simulink model "TST_CnvSet_Trq2Q"  (R2016b)
settings: Solver=FixedStepDiscrete  StartTime=0.0  StopTime=0.02  FixedStep=sampleTime  RelTol=1e-3
values from neighbouring files (symbols this model uses):
  testCase = 1    [initTST_CnvSet_Trq2Q_001.m]    (also in initTST_CnvSet_Trq2Q_002.m = 2; initTST_CnvSet_Trq2Q_003.m = 3)
libraries: simulink x31, UnitTest_Lib x27
settings Model: Creator=zhengjinyan  LastModifiedBy=zhengjinyan
settings DebuggingCC: SignalRangeChecking=error

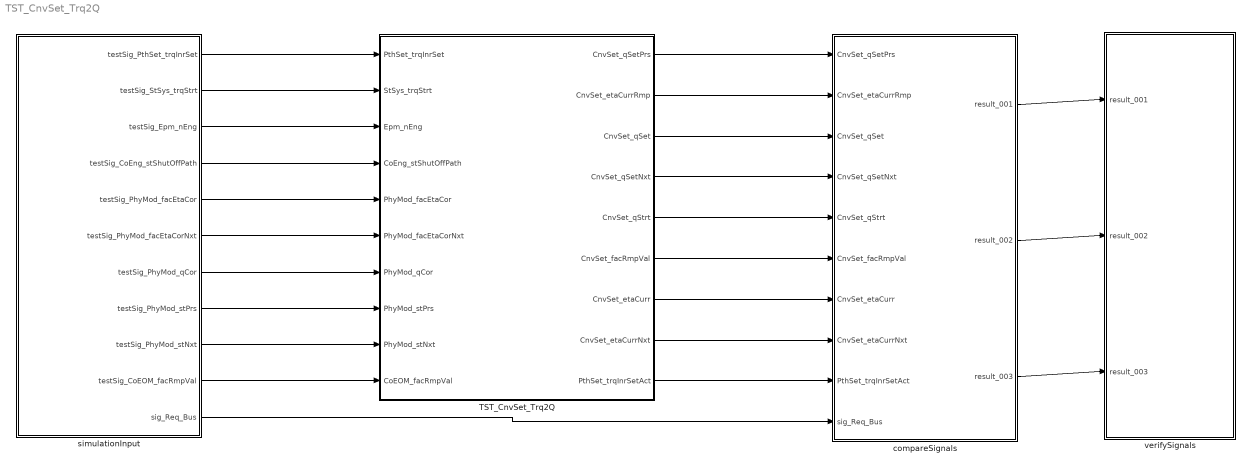
== system TST_CnvSet_Trq2Q ==
  TST_CnvSet_Trq2Q : Subsystem
  compareSignals : Subsystem
  simulationInput : Subsystem
  verifySignals : Subsystem
  wires:
  simulationInput/1(testSig_PthSet_trqInrSet) -> TST_CnvSet_Trq2Q/1(PthSet_trqInrSet)
  simulationInput/2(testSig_StSys_trqStrt) -> TST_CnvSet_Trq2Q/2(StSys_trqStrt)
  simulationInput/3(testSig_Epm_nEng) -> TST_CnvSet_Trq2Q/3(Epm_nEng)
  simulationInput/4(testSig_CoEng_stShutOffPath) -> TST_CnvSet_Trq2Q/4(CoEng_stShutOffPath)
  simulationInput/5(testSig_PhyMod_facEtaCor) -> TST_CnvSet_Trq2Q/5(PhyMod_facEtaCor)
  simulationInput/6(testSig_PhyMod_facEtaCorNxt) -> TST_CnvSet_Trq2Q/6(PhyMod_facEtaCorNxt)
  simulationInput/7(testSig_PhyMod_qCor) -> TST_CnvSet_Trq2Q/7(PhyMod_qCor)
  simulationInput/8(testSig_PhyMod_stPrs) -> TST_CnvSet_Trq2Q/8(PhyMod_stPrs)
  simulationInput/9(testSig_PhyMod_stNxt) -> TST_CnvSet_Trq2Q/9(PhyMod_stNxt)
  simulationInput/10(testSig_CoEOM_facRmpVal) -> TST_CnvSet_Trq2Q/10(CoEOM_facRmpVal)
  TST_CnvSet_Trq2Q/1(CnvSet_qSetPrs) -> compareSignals/1(CnvSet_qSetPrs)
  TST_CnvSet_Trq2Q/2(CnvSet_etaCurrRmp) -> compareSignals/2(CnvSet_etaCurrRmp)
  TST_CnvSet_Trq2Q/3(CnvSet_qSet) -> compareSignals/3(CnvSet_qSet)
  TST_CnvSet_Trq2Q/4(CnvSet_qSetNxt) -> compareSignals/4(CnvSet_qSetNxt)
  TST_CnvSet_Trq2Q/5(CnvSet_qStrt) -> compareSignals/5(CnvSet_qStrt)
  TST_CnvSet_Trq2Q/6(CnvSet_facRmpVal) -> compareSignals/6(CnvSet_facRmpVal)
  TST_CnvSet_Trq2Q/7(CnvSet_etaCurr) -> compareSignals/7(CnvSet_etaCurr)
  TST_CnvSet_Trq2Q/8(CnvSet_etaCurrNxt) -> compareSignals/8(CnvSet_etaCurrNxt)
  TST_CnvSet_Trq2Q/9(PthSet_trqInrSetAct) -> compareSignals/9(PthSet_trqInrSetAct)
  simulationInput/11(sig_Req_Bus) -> compareSignals/10(sig_Req_Bus)
  compareSignals/1(result_001) -> verifySignals/1(result_001)
  compareSignals/2(result_002) -> verifySignals/2(result_002)
  compareSignals/3(result_003) -> verifySignals/3(result_003)

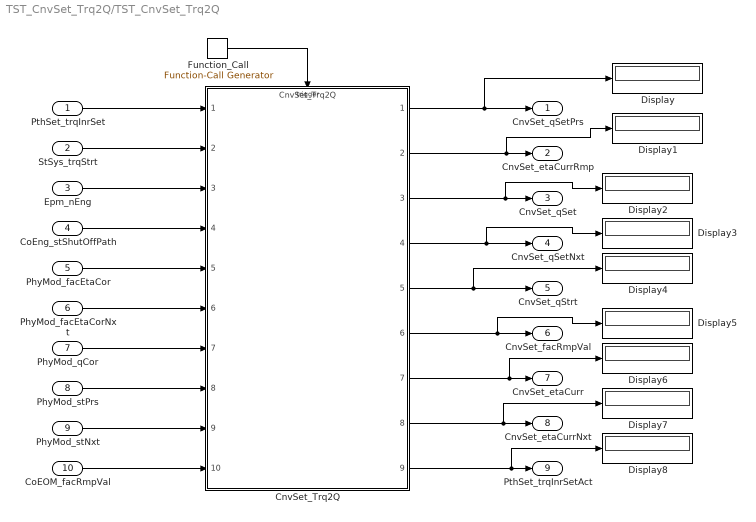
== system TST_CnvSet_Trq2Q/TST_CnvSet_Trq2Q ==
  PthSet_trqInrSet : Inport
  StSys_trqStrt : Inport  Port=2
  Epm_nEng : Inport  Port=3
  CoEng_stShutOffPath : Inport  Port=4
  PhyMod_facEtaCor : Inport  Port=5
  PhyMod_facEtaCorNxt : Inport  Port=6
  PhyMod_qCor : Inport  Port=7
  PhyMod_stPrs : Inport  Port=8
  PhyMod_stNxt : Inport  Port=9
  CoEOM_facRmpVal : Inport  Port=10
  CnvSet_Trq2Q : ModelReference  ModelNameDialog=CnvSet_Trq2Q  SimulationMode=Normal  ModelReferenceVersion=1.56  TriggerPortName=function  TriggerPortTriggerType=function-call  TriggerPortStatesWhenEnabling=held
  Display{,1..8} (9 alike) : Display
  Function_Call : simulink/Ports & Subsystems/Function-Call Generator  sample_time=sampleTime  numberOfIterations=1
  CnvSet_qSetPrs : Outport
  CnvSet_etaCurrRmp : Outport  Port=2
  CnvSet_qSet : Outport  Port=3
  CnvSet_qSetNxt : Outport  Port=4
  CnvSet_qStrt : Outport  Port=5
  CnvSet_facRmpVal : Outport  Port=6
  CnvSet_etaCurr : Outport  Port=7
  CnvSet_etaCurrNxt : Outport  Port=8
  PthSet_trqInrSetAct : Outport  Port=9
  wires:
  Function_Call/1 -> CnvSet_Trq2Q/Trigger
  PthSet_trqInrSet/1 -> CnvSet_Trq2Q/1
  StSys_trqStrt/1 -> CnvSet_Trq2Q/2
  Epm_nEng/1 -> CnvSet_Trq2Q/3
  CoEng_stShutOffPath/1 -> CnvSet_Trq2Q/4
  PhyMod_facEtaCor/1 -> CnvSet_Trq2Q/5
  PhyMod_facEtaCorNxt/1 -> CnvSet_Trq2Q/6
  PhyMod_qCor/1 -> CnvSet_Trq2Q/7
  PhyMod_stPrs/1 -> CnvSet_Trq2Q/8
  PhyMod_stNxt/1 -> CnvSet_Trq2Q/9
  CoEOM_facRmpVal/1 -> CnvSet_Trq2Q/10
  CnvSet_Trq2Q/1 -> Display/1, CnvSet_qSetPrs/1
  CnvSet_Trq2Q/2 -> Display1/1, CnvSet_etaCurrRmp/1
  CnvSet_Trq2Q/3 -> Display2/1, CnvSet_qSet/1
  CnvSet_Trq2Q/4 -> Display3/1, CnvSet_qSetNxt/1
  CnvSet_Trq2Q/5 -> Display4/1, CnvSet_qStrt/1
  CnvSet_Trq2Q/6 -> Display5/1, CnvSet_facRmpVal/1
  CnvSet_Trq2Q/7 -> Display6/1, CnvSet_etaCurr/1
  CnvSet_Trq2Q/9 -> Display8/1, PthSet_trqInrSetAct/1
  CnvSet_Trq2Q/8 -> Display7/1, CnvSet_etaCurrNxt/1

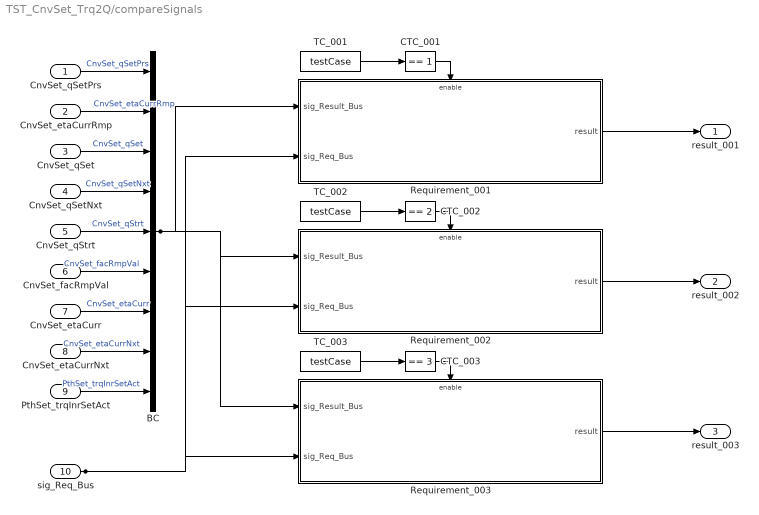
== system TST_CnvSet_Trq2Q/compareSignals ==
  CnvSet_qSetPrs : Inport
  CnvSet_etaCurrRmp : Inport  Port=2
  CnvSet_qSet : Inport  Port=3
  CnvSet_qSetNxt : Inport  Port=4
  CnvSet_qStrt : Inport  Port=5
  CnvSet_facRmpVal : Inport  Port=6
  CnvSet_etaCurr : Inport  Port=7
  CnvSet_etaCurrNxt : Inport  Port=8
  PthSet_trqInrSetAct : Inport  Port=9
  sig_Req_Bus : Inport  Port=10
  BC : BusCreator  Inputs=9
  CTC_001 : simulink/Logic and Bit Operations/Compare To Constant  relop===  const=1  OutDataTypeStr=boolean
  CTC_002 : simulink/Logic and Bit Operations/Compare To Constant  relop===  const=2  OutDataTypeStr=boolean
  CTC_003 : simulink/Logic and Bit Operations/Compare To Constant  relop===  const=3  OutDataTypeStr=boolean
  Requirement_001 : Subsystem
  Requirement_002 : Subsystem
  Requirement_003 : Subsystem
  TC_001 : Constant  Value=testCase
  TC_002 : Constant  Value=testCase
  TC_003 : Constant  Value=testCase
  result_001 : Outport
  result_002 : Outport  Port=2
  result_003 : Outport  Port=3
  wires:
  CnvSet_qSetPrs/1 -> BC/1  "CnvSet_qSetPrs"
  CnvSet_etaCurrRmp/1 -> BC/2  "CnvSet_etaCurrRmp"
  CnvSet_qSet/1 -> BC/3  "CnvSet_qSet"
  CnvSet_qSetNxt/1 -> BC/4  "CnvSet_qSetNxt"
  CnvSet_qStrt/1 -> BC/5  "CnvSet_qStrt"
  CnvSet_facRmpVal/1 -> BC/6  "CnvSet_facRmpVal"
  CnvSet_etaCurr/1 -> BC/7  "CnvSet_etaCurr"
  CnvSet_etaCurrNxt/1 -> BC/8  "CnvSet_etaCurrNxt"
  PthSet_trqInrSetAct/1 -> BC/9  "PthSet_trqInrSetAct"
  TC_001/1 -> CTC_001/1
  CTC_001/1 -> Requirement_001/Enable
  sig_Req_Bus/1 -> Requirement_001/2(sig_Req_Bus), Requirement_002/2(sig_Req_Bus), Requirement_003/2(sig_Req_Bus)
  BC/1 -> Requirement_001/1(sig_Result_Bus), Requirement_002/1(sig_Result_Bus), Requirement_003/1(sig_Result_Bus)
  Requirement_001/1(result) -> result_001/1
  TC_002/1 -> CTC_002/1
  CTC_002/1 -> Requirement_002/Enable
  Requirement_002/1(result) -> result_002/1
  TC_003/1 -> CTC_003/1
  CTC_003/1 -> Requirement_003/Enable
  Requirement_003/1(result) -> result_003/1

== system TST_CnvSet_Trq2Q/simulationInput ==
  BS : BusSelector  OutputSignals=testSig_PthSet_trqInrSet,testSig_StSys_trqStrt,testSig_Epm_nEng,testSig_CoEng_stShutOffPath,testSig_PhyMod_facEtaCor,testSig_PhyMod_facEtaCorNxt,testSig_PhyMod_qCor,testSig_PhyMod_stPrs,testSig_PhyMod_stNxt,testSig_CoEOM_facRmpVal
  MPSw : MultiPortSwitch  SaturateOnIntegerOverflow=on  InputSameDT=on
  TestCase : Constant  Value=testCase
  testSignals_R001 : Subsystem
  testSignals_R002 : Subsystem
  testSignals_R003 : Subsystem
  testSig_PthSet_trqInrSet : Outport
  testSig_StSys_trqStrt : Outport  Port=2
  testSig_Epm_nEng : Outport  Port=3
  testSig_CoEng_stShutOffPath : Outport  Port=4
  testSig_PhyMod_facEtaCor : Outport  Port=5
  testSig_PhyMod_facEtaCorNxt : Outport  Port=6
  testSig_PhyMod_qCor : Outport  Port=7
  testSig_PhyMod_stPrs : Outport  Port=8
  testSig_PhyMod_stNxt : Outport  Port=9
  testSig_CoEOM_facRmpVal : Outport  Port=10
  sig_Req_Bus : Outport  Port=11
  wires:
  BS/1 -> testSig_PthSet_trqInrSet/1  "<testSig_PthSet_trqInrSet>"
  BS/2 -> testSig_StSys_trqStrt/1  "<testSig_StSys_trqStrt>"
  BS/3 -> testSig_Epm_nEng/1  "<testSig_Epm_nEng>"
  BS/4 -> testSig_CoEng_stShutOffPath/1  "<testSig_CoEng_stShutOffPath>"
  BS/5 -> testSig_PhyMod_facEtaCor/1  "<testSig_PhyMod_facEtaCor>"
  BS/6 -> testSig_PhyMod_facEtaCorNxt/1  "<testSig_PhyMod_facEtaCorNxt>"
  BS/7 -> testSig_PhyMod_qCor/1  "<testSig_PhyMod_qCor>"
  BS/8 -> testSig_PhyMod_stPrs/1  "<testSig_PhyMod_stPrs>"
  BS/9 -> testSig_PhyMod_stNxt/1  "<testSig_PhyMod_stNxt>"
  BS/10 -> testSig_CoEOM_facRmpVal/1  "<testSig_CoEOM_facRmpVal>"
  MPSw/1 -> BS/1, sig_Req_Bus/1
  TestCase/1 -> MPSw/1
  testSignals_R001/1(testSignals) -> MPSw/2
  testSignals_R002/1(testSignals) -> MPSw/3
  testSignals_R003/1(testSignals) -> MPSw/4

== system TST_CnvSet_Trq2Q/verifySignals ==
  result_001 : Inport
  result_002 : Inport  Port=2
  result_003 : Inport  Port=3
  Assertion_001 : Assertion  Enabled=off
  Assertion_002 : Assertion  Enabled=off
  Assertion_003 : Assertion  Enabled=off
  wires:
  result_001/1 -> Assertion_001/1
  result_002/1 -> Assertion_002/1
  result_003/1 -> Assertion_003/1

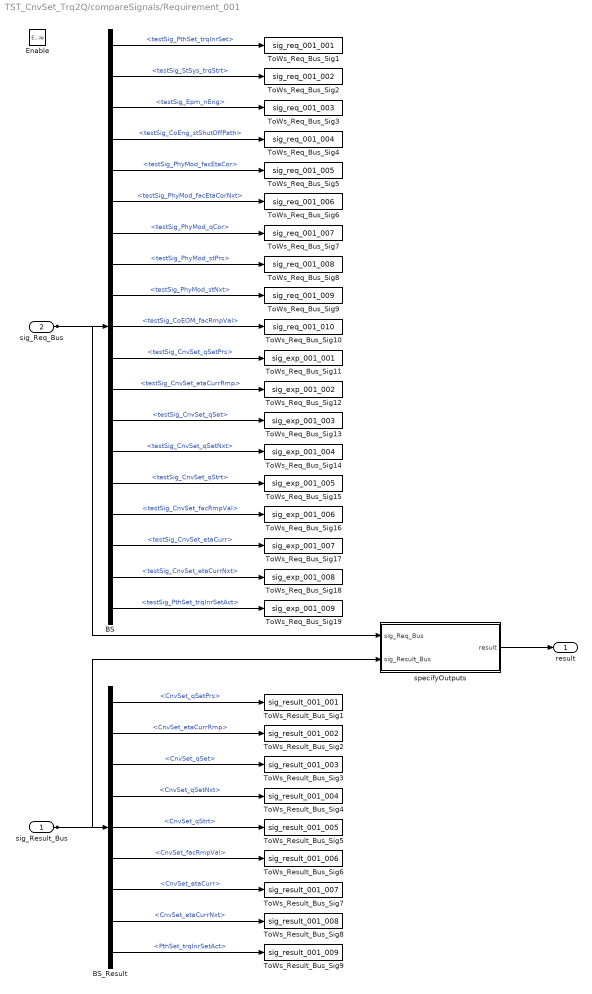
== system TST_CnvSet_Trq2Q/compareSignals/Requirement_001 ==
  sig_Result_Bus : Inport
  sig_Req_Bus : Inport  Port=2
  Enable : EnablePort
  BS : BusSelector  OutputSignals=testSig_PthSet_trqInrSet,testSig_StSys_trqStrt,testSig_Epm_nEng,testSig_CoEng_stShutOffPath,testSig_PhyMod_facEtaCor,testSig_PhyMod_facEtaCorNxt,testSig_PhyMod_qCor,testSig_PhyMod_stPrs,testSig_PhyMod_stNxt,testSig_CoEOM_facRmpVal,testSig_CnvSet_qSetPrs,testSig_CnvSet_etaCurrRmp,testSig_CnvSet_qSet,testSig_CnvSet_qSetNxt,testSig_CnvSet_qStrt,testSig_CnvSet_facRmpVal,testSig_CnvSet_etaCurr,testSig_CnvSet_etaCurrNxt,testSig_PthSet_trqInrSetAct
  BS_Result : BusSelector  OutputSignals=CnvSet_qSetPrs,CnvSet_etaCurrRmp,CnvSet_qSet,CnvSet_qSetNxt,CnvSet_qStrt,CnvSet_facRmpVal,CnvSet_etaCurr,CnvSet_etaCurrNxt,PthSet_trqInrSetAct
  ToWs_Req_Bus_Sig1 : ToWorkspace  VariableName=sig_req_001_001  SaveFormat=Structure With Time
  ToWs_Req_Bus_Sig10 : ToWorkspace  VariableName=sig_req_001_010  SaveFormat=Structure With Time
  ToWs_Req_Bus_Sig11 : ToWorkspace  VariableName=sig_exp_001_001  SaveFormat=Structure With Time
  ToWs_Req_Bus_Sig12 : ToWorkspace  VariableName=sig_exp_001_002  SaveFormat=Structure With Time
  ToWs_Req_Bus_Sig13 : ToWorkspace  VariableName=sig_exp_001_003  SaveFormat=Structure With Time
  ToWs_Req_Bus_Sig14 : ToWorkspace  VariableName=sig_exp_001_004  SaveFormat=Structure With Time
  ToWs_Req_Bus_Sig15 : ToWorkspace  VariableName=sig_exp_001_005  SaveFormat=Structure With Time
  ToWs_Req_Bus_Sig16 : ToWorkspace  VariableName=sig_exp_001_006  SaveFormat=Structure With Time
  ToWs_Req_Bus_Sig17 : ToWorkspace  VariableName=sig_exp_001_007  SaveFormat=Structure With Time
  ToWs_Req_Bus_Sig18 : ToWorkspace  VariableName=sig_exp_001_008  SaveFormat=Structure With Time
  ToWs_Req_Bus_Sig19 : ToWorkspace  VariableName=sig_exp_001_009  SaveFormat=Structure With Time
  ToWs_Req_Bus_Sig2 : ToWorkspace  VariableName=sig_req_001_002  SaveFormat=Structure With Time
  ToWs_Req_Bus_Sig3 : ToWorkspace  VariableName=sig_req_001_003  SaveFormat=Structure With Time
  ToWs_Req_Bus_Sig4 : ToWorkspace  VariableName=sig_req_001_004  SaveFormat=Structure With Time
  ToWs_Req_Bus_Sig5 : ToWorkspace  VariableName=sig_req_001_005  SaveFormat=Structure With Time
  ToWs_Req_Bus_Sig6 : ToWorkspace  VariableName=sig_req_001_006  SaveFormat=Structure With Time
  ToWs_Req_Bus_Sig7 : ToWorkspace  VariableName=sig_req_001_007  SaveFormat=Structure With Time
  ToWs_Req_Bus_Sig8 : ToWorkspace  VariableName=sig_req_001_008  SaveFormat=Structure With Time
  ToWs_Req_Bus_Sig9 : ToWorkspace  VariableName=sig_req_001_009  SaveFormat=Structure With Time
  ToWs_Result_Bus_Sig1 : ToWorkspace  VariableName=sig_result_001_001  SaveFormat=Structure With Time
  ToWs_Result_Bus_Sig2 : ToWorkspace  VariableName=sig_result_001_002  SaveFormat=Structure With Time
  ToWs_Result_Bus_Sig3 : ToWorkspace  VariableName=sig_result_001_003  SaveFormat=Structure With Time
  ToWs_Result_Bus_Sig4 : ToWorkspace  VariableName=sig_result_001_004  SaveFormat=Structure With Time
  ToWs_Result_Bus_Sig5 : ToWorkspace  VariableName=sig_result_001_005  SaveFormat=Structure With Time
  ToWs_Result_Bus_Sig6 : ToWorkspace  VariableName=sig_result_001_006  SaveFormat=Structure With Time
  ToWs_Result_Bus_Sig7 : ToWorkspace  VariableName=sig_result_001_007  SaveFormat=Structure With Time
  ToWs_Result_Bus_Sig8 : ToWorkspace  VariableName=sig_result_001_008  SaveFormat=Structure With Time
  ToWs_Result_Bus_Sig9 : ToWorkspace  VariableName=sig_result_001_009  SaveFormat=Structure With Time
  specifyOutputs : Subsystem
  result : Outport
  wires:
  sig_Req_Bus/1 -> BS/1, specifyOutputs/1(sig_Req_Bus)
  BS/1 -> ToWs_Req_Bus_Sig1/1  "<testSig_PthSet_trqInrSet>"
  BS/2 -> ToWs_Req_Bus_Sig2/1  "<testSig_StSys_trqStrt>"
  BS/3 -> ToWs_Req_Bus_Sig3/1  "<testSig_Epm_nEng>"
  BS/4 -> ToWs_Req_Bus_Sig4/1  "<testSig_CoEng_stShutOffPath>"
  BS/5 -> ToWs_Req_Bus_Sig5/1  "<testSig_PhyMod_facEtaCor>"
  BS/6 -> ToWs_Req_Bus_Sig6/1  "<testSig_PhyMod_facEtaCorNxt>"
  BS/7 -> ToWs_Req_Bus_Sig7/1  "<testSig_PhyMod_qCor>"
  BS/8 -> ToWs_Req_Bus_Sig8/1  "<testSig_PhyMod_stPrs>"
  BS/9 -> ToWs_Req_Bus_Sig9/1  "<testSig_PhyMod_stNxt>"
  BS/10 -> ToWs_Req_Bus_Sig10/1  "<testSig_CoEOM_facRmpVal>"
  BS/11 -> ToWs_Req_Bus_Sig11/1  "<testSig_CnvSet_qSetPrs>"
  BS/12 -> ToWs_Req_Bus_Sig12/1  "<testSig_CnvSet_etaCurrRmp>"
  BS/13 -> ToWs_Req_Bus_Sig13/1  "<testSig_CnvSet_qSet>"
  BS/14 -> ToWs_Req_Bus_Sig14/1  "<testSig_CnvSet_qSetNxt>"
  BS/15 -> ToWs_Req_Bus_Sig15/1  "<testSig_CnvSet_qStrt>"
  BS/16 -> ToWs_Req_Bus_Sig16/1  "<testSig_CnvSet_facRmpVal>"
  BS/17 -> ToWs_Req_Bus_Sig17/1  "<testSig_CnvSet_etaCurr>"
  BS/18 -> ToWs_Req_Bus_Sig18/1  "<testSig_CnvSet_etaCurrNxt>"
  BS/19 -> ToWs_Req_Bus_Sig19/1  "<testSig_PthSet_trqInrSetAct>"
  sig_Result_Bus/1 -> BS_Result/1, specifyOutputs/2(sig_Result_Bus)
  BS_Result/1 -> ToWs_Result_Bus_Sig1/1  "<CnvSet_qSetPrs>"
  BS_Result/2 -> ToWs_Result_Bus_Sig2/1  "<CnvSet_etaCurrRmp>"
  BS_Result/3 -> ToWs_Result_Bus_Sig3/1  "<CnvSet_qSet>"
  BS_Result/4 -> ToWs_Result_Bus_Sig4/1  "<CnvSet_qSetNxt>"
  BS_Result/5 -> ToWs_Result_Bus_Sig5/1  "<CnvSet_qStrt>"
  BS_Result/6 -> ToWs_Result_Bus_Sig6/1  "<CnvSet_facRmpVal>"
  BS_Result/7 -> ToWs_Result_Bus_Sig7/1  "<CnvSet_etaCurr>"
  BS_Result/8 -> ToWs_Result_Bus_Sig8/1  "<CnvSet_etaCurrNxt>"
  BS_Result/9 -> ToWs_Result_Bus_Sig9/1  "<PthSet_trqInrSetAct>"
  specifyOutputs/1(result) -> result/1

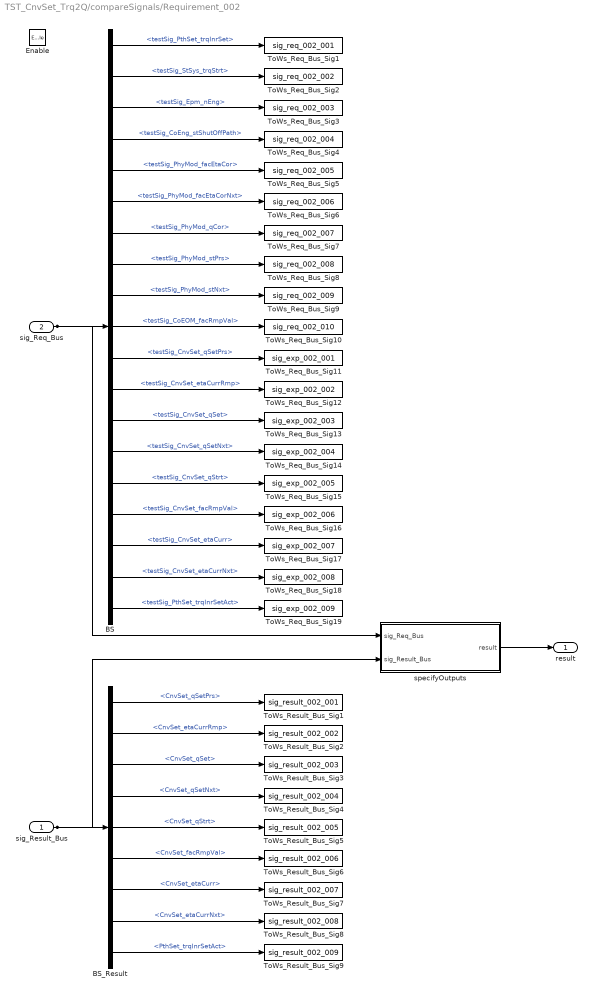
== system TST_CnvSet_Trq2Q/compareSignals/Requirement_002 ==
  sig_Result_Bus : Inport
  sig_Req_Bus : Inport  Port=2
  Enable : EnablePort
  BS : BusSelector  OutputSignals=testSig_PthSet_trqInrSet,testSig_StSys_trqStrt,testSig_Epm_nEng,testSig_CoEng_stShutOffPath,testSig_PhyMod_facEtaCor,testSig_PhyMod_facEtaCorNxt,testSig_PhyMod_qCor,testSig_PhyMod_stPrs,testSig_PhyMod_stNxt,testSig_CoEOM_facRmpVal,testSig_CnvSet_qSetPrs,testSig_CnvSet_etaCurrRmp,testSig_CnvSet_qSet,testSig_CnvSet_qSetNxt,testSig_CnvSet_qStrt,testSig_CnvSet_facRmpVal,testSig_CnvSet_etaCurr,testSig_CnvSet_etaCurrNxt,testSig_PthSet_trqInrSetAct
  BS_Result : BusSelector  OutputSignals=CnvSet_qSetPrs,CnvSet_etaCurrRmp,CnvSet_qSet,CnvSet_qSetNxt,CnvSet_qStrt,CnvSet_facRmpVal,CnvSet_etaCurr,CnvSet_etaCurrNxt,PthSet_trqInrSetAct
  ToWs_Req_Bus_Sig1 : ToWorkspace  VariableName=sig_req_002_001  SaveFormat=Structure With Time
  ToWs_Req_Bus_Sig10 : ToWorkspace  VariableName=sig_req_002_010  SaveFormat=Structure With Time
  ToWs_Req_Bus_Sig11 : ToWorkspace  VariableName=sig_exp_002_001  SaveFormat=Structure With Time
  ToWs_Req_Bus_Sig12 : ToWorkspace  VariableName=sig_exp_002_002  SaveFormat=Structure With Time
  ToWs_Req_Bus_Sig13 : ToWorkspace  VariableName=sig_exp_002_003  SaveFormat=Structure With Time
  ToWs_Req_Bus_Sig14 : ToWorkspace  VariableName=sig_exp_002_004  SaveFormat=Structure With Time
  ToWs_Req_Bus_Sig15 : ToWorkspace  VariableName=sig_exp_002_005  SaveFormat=Structure With Time
  ToWs_Req_Bus_Sig16 : ToWorkspace  VariableName=sig_exp_002_006  SaveFormat=Structure With Time
  ToWs_Req_Bus_Sig17 : ToWorkspace  VariableName=sig_exp_002_007  SaveFormat=Structure With Time
  ToWs_Req_Bus_Sig18 : ToWorkspace  VariableName=sig_exp_002_008  SaveFormat=Structure With Time
  ToWs_Req_Bus_Sig19 : ToWorkspace  VariableName=sig_exp_002_009  SaveFormat=Structure With Time
  ToWs_Req_Bus_Sig2 : ToWorkspace  VariableName=sig_req_002_002  SaveFormat=Structure With Time
  ToWs_Req_Bus_Sig3 : ToWorkspace  VariableName=sig_req_002_003  SaveFormat=Structure With Time
  ToWs_Req_Bus_Sig4 : ToWorkspace  VariableName=sig_req_002_004  SaveFormat=Structure With Time
  ToWs_Req_Bus_Sig5 : ToWorkspace  VariableName=sig_req_002_005  SaveFormat=Structure With Time
  ToWs_Req_Bus_Sig6 : ToWorkspace  VariableName=sig_req_002_006  SaveFormat=Structure With Time
  ToWs_Req_Bus_Sig7 : ToWorkspace  VariableName=sig_req_002_007  SaveFormat=Structure With Time
  ToWs_Req_Bus_Sig8 : ToWorkspace  VariableName=sig_req_002_008  SaveFormat=Structure With Time
  ToWs_Req_Bus_Sig9 : ToWorkspace  VariableName=sig_req_002_009  SaveFormat=Structure With Time
  ToWs_Result_Bus_Sig1 : ToWorkspace  VariableName=sig_result_002_001  SaveFormat=Structure With Time
  ToWs_Result_Bus_Sig2 : ToWorkspace  VariableName=sig_result_002_002  SaveFormat=Structure With Time
  ToWs_Result_Bus_Sig3 : ToWorkspace  VariableName=sig_result_002_003  SaveFormat=Structure With Time
  ToWs_Result_Bus_Sig4 : ToWorkspace  VariableName=sig_result_002_004  SaveFormat=Structure With Time
  ToWs_Result_Bus_Sig5 : ToWorkspace  VariableName=sig_result_002_005  SaveFormat=Structure With Time
  ToWs_Result_Bus_Sig6 : ToWorkspace  VariableName=sig_result_002_006  SaveFormat=Structure With Time
  ToWs_Result_Bus_Sig7 : ToWorkspace  VariableName=sig_result_002_007  SaveFormat=Structure With Time
  ToWs_Result_Bus_Sig8 : ToWorkspace  VariableName=sig_result_002_008  SaveFormat=Structure With Time
  ToWs_Result_Bus_Sig9 : ToWorkspace  VariableName=sig_result_002_009  SaveFormat=Structure With Time
  specifyOutputs : Subsystem
  result : Outport
  wires:
  sig_Req_Bus/1 -> BS/1, specifyOutputs/1(sig_Req_Bus)
  BS/1 -> ToWs_Req_Bus_Sig1/1  "<testSig_PthSet_trqInrSet>"
  BS/2 -> ToWs_Req_Bus_Sig2/1  "<testSig_StSys_trqStrt>"
  BS/3 -> ToWs_Req_Bus_Sig3/1  "<testSig_Epm_nEng>"
  BS/4 -> ToWs_Req_Bus_Sig4/1  "<testSig_CoEng_stShutOffPath>"
  BS/5 -> ToWs_Req_Bus_Sig5/1  "<testSig_PhyMod_facEtaCor>"
  BS/6 -> ToWs_Req_Bus_Sig6/1  "<testSig_PhyMod_facEtaCorNxt>"
  BS/7 -> ToWs_Req_Bus_Sig7/1  "<testSig_PhyMod_qCor>"
  BS/8 -> ToWs_Req_Bus_Sig8/1  "<testSig_PhyMod_stPrs>"
  BS/9 -> ToWs_Req_Bus_Sig9/1  "<testSig_PhyMod_stNxt>"
  BS/10 -> ToWs_Req_Bus_Sig10/1  "<testSig_CoEOM_facRmpVal>"
  BS/11 -> ToWs_Req_Bus_Sig11/1  "<testSig_CnvSet_qSetPrs>"
  BS/12 -> ToWs_Req_Bus_Sig12/1  "<testSig_CnvSet_etaCurrRmp>"
  BS/13 -> ToWs_Req_Bus_Sig13/1  "<testSig_CnvSet_qSet>"
  BS/14 -> ToWs_Req_Bus_Sig14/1  "<testSig_CnvSet_qSetNxt>"
  BS/15 -> ToWs_Req_Bus_Sig15/1  "<testSig_CnvSet_qStrt>"
  BS/16 -> ToWs_Req_Bus_Sig16/1  "<testSig_CnvSet_facRmpVal>"
  BS/17 -> ToWs_Req_Bus_Sig17/1  "<testSig_CnvSet_etaCurr>"
  BS/18 -> ToWs_Req_Bus_Sig18/1  "<testSig_CnvSet_etaCurrNxt>"
  BS/19 -> ToWs_Req_Bus_Sig19/1  "<testSig_PthSet_trqInrSetAct>"
  sig_Result_Bus/1 -> BS_Result/1, specifyOutputs/2(sig_Result_Bus)
  BS_Result/1 -> ToWs_Result_Bus_Sig1/1  "<CnvSet_qSetPrs>"
  BS_Result/2 -> ToWs_Result_Bus_Sig2/1  "<CnvSet_etaCurrRmp>"
  BS_Result/3 -> ToWs_Result_Bus_Sig3/1  "<CnvSet_qSet>"
  BS_Result/4 -> ToWs_Result_Bus_Sig4/1  "<CnvSet_qSetNxt>"
  BS_Result/5 -> ToWs_Result_Bus_Sig5/1  "<CnvSet_qStrt>"
  BS_Result/6 -> ToWs_Result_Bus_Sig6/1  "<CnvSet_facRmpVal>"
  BS_Result/7 -> ToWs_Result_Bus_Sig7/1  "<CnvSet_etaCurr>"
  BS_Result/8 -> ToWs_Result_Bus_Sig8/1  "<CnvSet_etaCurrNxt>"
  BS_Result/9 -> ToWs_Result_Bus_Sig9/1  "<PthSet_trqInrSetAct>"
  specifyOutputs/1(result) -> result/1

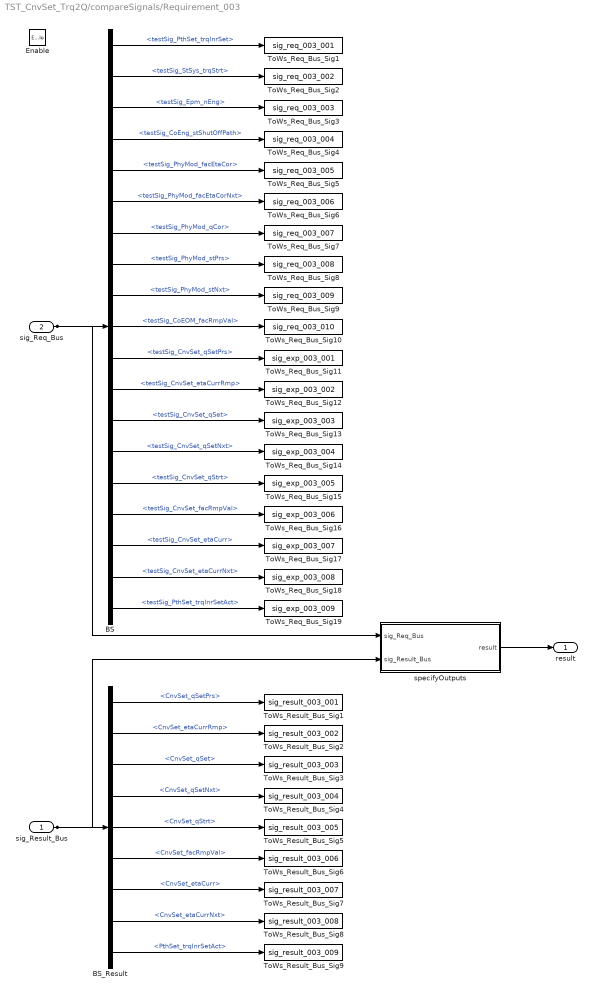
== system TST_CnvSet_Trq2Q/compareSignals/Requirement_003 ==
  sig_Result_Bus : Inport
  sig_Req_Bus : Inport  Port=2
  Enable : EnablePort
  BS : BusSelector  OutputSignals=testSig_PthSet_trqInrSet,testSig_StSys_trqStrt,testSig_Epm_nEng,testSig_CoEng_stShutOffPath,testSig_PhyMod_facEtaCor,testSig_PhyMod_facEtaCorNxt,testSig_PhyMod_qCor,testSig_PhyMod_stPrs,testSig_PhyMod_stNxt,testSig_CoEOM_facRmpVal,testSig_CnvSet_qSetPrs,testSig_CnvSet_etaCurrRmp,testSig_CnvSet_qSet,testSig_CnvSet_qSetNxt,testSig_CnvSet_qStrt,testSig_CnvSet_facRmpVal,testSig_CnvSet_etaCurr,testSig_CnvSet_etaCurrNxt,testSig_PthSet_trqInrSetAct
  BS_Result : BusSelector  OutputSignals=CnvSet_qSetPrs,CnvSet_etaCurrRmp,CnvSet_qSet,CnvSet_qSetNxt,CnvSet_qStrt,CnvSet_facRmpVal,CnvSet_etaCurr,CnvSet_etaCurrNxt,PthSet_trqInrSetAct
  ToWs_Req_Bus_Sig1 : ToWorkspace  VariableName=sig_req_003_001  SaveFormat=Structure With Time
  ToWs_Req_Bus_Sig10 : ToWorkspace  VariableName=sig_req_003_010  SaveFormat=Structure With Time
  ToWs_Req_Bus_Sig11 : ToWorkspace  VariableName=sig_exp_003_001  SaveFormat=Structure With Time
  ToWs_Req_Bus_Sig12 : ToWorkspace  VariableName=sig_exp_003_002  SaveFormat=Structure With Time
  ToWs_Req_Bus_Sig13 : ToWorkspace  VariableName=sig_exp_003_003  SaveFormat=Structure With Time
  ToWs_Req_Bus_Sig14 : ToWorkspace  VariableName=sig_exp_003_004  SaveFormat=Structure With Time
  ToWs_Req_Bus_Sig15 : ToWorkspace  VariableName=sig_exp_003_005  SaveFormat=Structure With Time
  ToWs_Req_Bus_Sig16 : ToWorkspace  VariableName=sig_exp_003_006  SaveFormat=Structure With Time
  ToWs_Req_Bus_Sig17 : ToWorkspace  VariableName=sig_exp_003_007  SaveFormat=Structure With Time
  ToWs_Req_Bus_Sig18 : ToWorkspace  VariableName=sig_exp_003_008  SaveFormat=Structure With Time
  ToWs_Req_Bus_Sig19 : ToWorkspace  VariableName=sig_exp_003_009  SaveFormat=Structure With Time
  ToWs_Req_Bus_Sig2 : ToWorkspace  VariableName=sig_req_003_002  SaveFormat=Structure With Time
  ToWs_Req_Bus_Sig3 : ToWorkspace  VariableName=sig_req_003_003  SaveFormat=Structure With Time
  ToWs_Req_Bus_Sig4 : ToWorkspace  VariableName=sig_req_003_004  SaveFormat=Structure With Time
  ToWs_Req_Bus_Sig5 : ToWorkspace  VariableName=sig_req_003_005  SaveFormat=Structure With Time
  ToWs_Req_Bus_Sig6 : ToWorkspace  VariableName=sig_req_003_006  SaveFormat=Structure With Time
  ToWs_Req_Bus_Sig7 : ToWorkspace  VariableName=sig_req_003_007  SaveFormat=Structure With Time
  ToWs_Req_Bus_Sig8 : ToWorkspace  VariableName=sig_req_003_008  SaveFormat=Structure With Time
  ToWs_Req_Bus_Sig9 : ToWorkspace  VariableName=sig_req_003_009  SaveFormat=Structure With Time
  ToWs_Result_Bus_Sig1 : ToWorkspace  VariableName=sig_result_003_001  SaveFormat=Structure With Time
  ToWs_Result_Bus_Sig2 : ToWorkspace  VariableName=sig_result_003_002  SaveFormat=Structure With Time
  ToWs_Result_Bus_Sig3 : ToWorkspace  VariableName=sig_result_003_003  SaveFormat=Structure With Time
  ToWs_Result_Bus_Sig4 : ToWorkspace  VariableName=sig_result_003_004  SaveFormat=Structure With Time
  ToWs_Result_Bus_Sig5 : ToWorkspace  VariableName=sig_result_003_005  SaveFormat=Structure With Time
  ToWs_Result_Bus_Sig6 : ToWorkspace  VariableName=sig_result_003_006  SaveFormat=Structure With Time
  ToWs_Result_Bus_Sig7 : ToWorkspace  VariableName=sig_result_003_007  SaveFormat=Structure With Time
  ToWs_Result_Bus_Sig8 : ToWorkspace  VariableName=sig_result_003_008  SaveFormat=Structure With Time
  ToWs_Result_Bus_Sig9 : ToWorkspace  VariableName=sig_result_003_009  SaveFormat=Structure With Time
  specifyOutputs : Subsystem
  result : Outport
  wires:
  sig_Req_Bus/1 -> BS/1, specifyOutputs/1(sig_Req_Bus)
  BS/1 -> ToWs_Req_Bus_Sig1/1  "<testSig_PthSet_trqInrSet>"
  BS/2 -> ToWs_Req_Bus_Sig2/1  "<testSig_StSys_trqStrt>"
  BS/3 -> ToWs_Req_Bus_Sig3/1  "<testSig_Epm_nEng>"
  BS/4 -> ToWs_Req_Bus_Sig4/1  "<testSig_CoEng_stShutOffPath>"
  BS/5 -> ToWs_Req_Bus_Sig5/1  "<testSig_PhyMod_facEtaCor>"
  BS/6 -> ToWs_Req_Bus_Sig6/1  "<testSig_PhyMod_facEtaCorNxt>"
  BS/7 -> ToWs_Req_Bus_Sig7/1  "<testSig_PhyMod_qCor>"
  BS/8 -> ToWs_Req_Bus_Sig8/1  "<testSig_PhyMod_stPrs>"
  BS/9 -> ToWs_Req_Bus_Sig9/1  "<testSig_PhyMod_stNxt>"
  BS/10 -> ToWs_Req_Bus_Sig10/1  "<testSig_CoEOM_facRmpVal>"
  BS/11 -> ToWs_Req_Bus_Sig11/1  "<testSig_CnvSet_qSetPrs>"
  BS/12 -> ToWs_Req_Bus_Sig12/1  "<testSig_CnvSet_etaCurrRmp>"
  BS/13 -> ToWs_Req_Bus_Sig13/1  "<testSig_CnvSet_qSet>"
  BS/14 -> ToWs_Req_Bus_Sig14/1  "<testSig_CnvSet_qSetNxt>"
  BS/15 -> ToWs_Req_Bus_Sig15/1  "<testSig_CnvSet_qStrt>"
  BS/16 -> ToWs_Req_Bus_Sig16/1  "<testSig_CnvSet_facRmpVal>"
  BS/17 -> ToWs_Req_Bus_Sig17/1  "<testSig_CnvSet_etaCurr>"
  BS/18 -> ToWs_Req_Bus_Sig18/1  "<testSig_CnvSet_etaCurrNxt>"
  BS/19 -> ToWs_Req_Bus_Sig19/1  "<testSig_PthSet_trqInrSetAct>"
  sig_Result_Bus/1 -> BS_Result/1, specifyOutputs/2(sig_Result_Bus)
  BS_Result/1 -> ToWs_Result_Bus_Sig1/1  "<CnvSet_qSetPrs>"
  BS_Result/2 -> ToWs_Result_Bus_Sig2/1  "<CnvSet_etaCurrRmp>"
  BS_Result/3 -> ToWs_Result_Bus_Sig3/1  "<CnvSet_qSet>"
  BS_Result/4 -> ToWs_Result_Bus_Sig4/1  "<CnvSet_qSetNxt>"
  BS_Result/5 -> ToWs_Result_Bus_Sig5/1  "<CnvSet_qStrt>"
  BS_Result/6 -> ToWs_Result_Bus_Sig6/1  "<CnvSet_facRmpVal>"
  BS_Result/7 -> ToWs_Result_Bus_Sig7/1  "<CnvSet_etaCurr>"
  BS_Result/8 -> ToWs_Result_Bus_Sig8/1  "<CnvSet_etaCurrNxt>"
  BS_Result/9 -> ToWs_Result_Bus_Sig9/1  "<PthSet_trqInrSetAct>"
  specifyOutputs/1(result) -> result/1

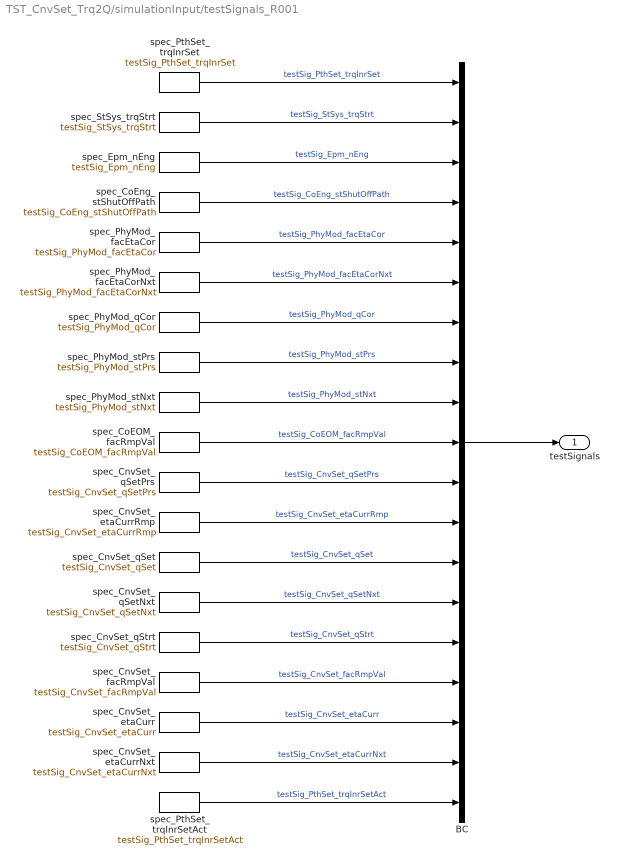
== system TST_CnvSet_Trq2Q/simulationInput/testSignals_R001 ==
  BC : BusCreator  Inputs=19
  spec_CnvSet_etaCurr : FromWorkspace  VariableName=testSig_CnvSet_etaCurr  Interpolate=off  OutputAfterFinalValue=Holding final value
  spec_CnvSet_etaCurrNxt : FromWorkspace  VariableName=testSig_CnvSet_etaCurrNxt  Interpolate=off  OutputAfterFinalValue=Holding final value
  spec_CnvSet_etaCurrRmp : FromWorkspace  VariableName=testSig_CnvSet_etaCurrRmp  Interpolate=off  OutputAfterFinalValue=Holding final value
  spec_CnvSet_facRmpVal : FromWorkspace  VariableName=testSig_CnvSet_facRmpVal  Interpolate=off  OutputAfterFinalValue=Holding final value
  spec_CnvSet_qSet : FromWorkspace  VariableName=testSig_CnvSet_qSet  Interpolate=off  OutputAfterFinalValue=Holding final value
  spec_CnvSet_qSetNxt : FromWorkspace  VariableName=testSig_CnvSet_qSetNxt  Interpolate=off  OutputAfterFinalValue=Holding final value
  spec_CnvSet_qSetPrs : FromWorkspace  VariableName=testSig_CnvSet_qSetPrs  Interpolate=off  OutputAfterFinalValue=Holding final value
  spec_CnvSet_qStrt : FromWorkspace  VariableName=testSig_CnvSet_qStrt  Interpolate=off  OutputAfterFinalValue=Holding final value
  spec_CoEOM_facRmpVal : FromWorkspace  VariableName=testSig_CoEOM_facRmpVal  Interpolate=off  OutputAfterFinalValue=Holding final value
  spec_CoEng_stShutOffPath : FromWorkspace  VariableName=testSig_CoEng_stShutOffPath  Interpolate=off  OutputAfterFinalValue=Holding final value
  spec_Epm_nEng : FromWorkspace  VariableName=testSig_Epm_nEng  Interpolate=off  OutputAfterFinalValue=Holding final value
  spec_PhyMod_facEtaCor : FromWorkspace  VariableName=testSig_PhyMod_facEtaCor  Interpolate=off  OutputAfterFinalValue=Holding final value
  spec_PhyMod_facEtaCorNxt : FromWorkspace  VariableName=testSig_PhyMod_facEtaCorNxt  Interpolate=off  OutputAfterFinalValue=Holding final value
  spec_PhyMod_qCor : FromWorkspace  VariableName=testSig_PhyMod_qCor  Interpolate=off  OutputAfterFinalValue=Holding final value
  spec_PhyMod_stNxt : FromWorkspace  VariableName=testSig_PhyMod_stNxt  Interpolate=off  OutputAfterFinalValue=Holding final value
  spec_PhyMod_stPrs : FromWorkspace  VariableName=testSig_PhyMod_stPrs  Interpolate=off  OutputAfterFinalValue=Holding final value
  spec_PthSet_trqInrSet : FromWorkspace  VariableName=testSig_PthSet_trqInrSet  Interpolate=off  OutputAfterFinalValue=Holding final value
  spec_PthSet_trqInrSetAct : FromWorkspace  VariableName=testSig_PthSet_trqInrSetAct  Interpolate=off  OutputAfterFinalValue=Holding final value
  spec_StSys_trqStrt : FromWorkspace  VariableName=testSig_StSys_trqStrt  Interpolate=off  OutputAfterFinalValue=Holding final value
  testSignals : Outport
  wires:
  BC/1 -> testSignals/1
  spec_PthSet_trqInrSet/1 -> BC/1  "testSig_PthSet_trqInrSet"
  spec_StSys_trqStrt/1 -> BC/2  "testSig_StSys_trqStrt"
  spec_Epm_nEng/1 -> BC/3  "testSig_Epm_nEng"
  spec_CoEng_stShutOffPath/1 -> BC/4  "testSig_CoEng_stShutOffPath"
  spec_PhyMod_facEtaCor/1 -> BC/5  "testSig_PhyMod_facEtaCor"
  spec_PhyMod_facEtaCorNxt/1 -> BC/6  "testSig_PhyMod_facEtaCorNxt"
  spec_PhyMod_qCor/1 -> BC/7  "testSig_PhyMod_qCor"
  spec_PhyMod_stPrs/1 -> BC/8  "testSig_PhyMod_stPrs"
  spec_PhyMod_stNxt/1 -> BC/9  "testSig_PhyMod_stNxt"
  spec_CoEOM_facRmpVal/1 -> BC/10  "testSig_CoEOM_facRmpVal"
  spec_CnvSet_qSetPrs/1 -> BC/11  "testSig_CnvSet_qSetPrs"
  spec_CnvSet_etaCurrRmp/1 -> BC/12  "testSig_CnvSet_etaCurrRmp"
  spec_CnvSet_qSet/1 -> BC/13  "testSig_CnvSet_qSet"
  spec_CnvSet_qSetNxt/1 -> BC/14  "testSig_CnvSet_qSetNxt"
  spec_CnvSet_qStrt/1 -> BC/15  "testSig_CnvSet_qStrt"
  spec_CnvSet_facRmpVal/1 -> BC/16  "testSig_CnvSet_facRmpVal"
  spec_CnvSet_etaCurr/1 -> BC/17  "testSig_CnvSet_etaCurr"
  spec_CnvSet_etaCurrNxt/1 -> BC/18  "testSig_CnvSet_etaCurrNxt"
  spec_PthSet_trqInrSetAct/1 -> BC/19  "testSig_PthSet_trqInrSetAct"

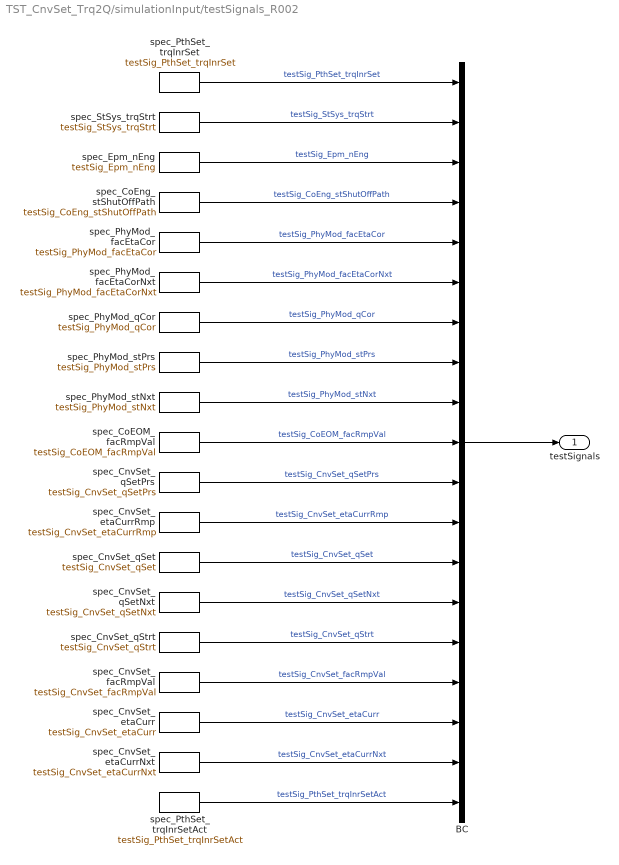
== system TST_CnvSet_Trq2Q/simulationInput/testSignals_R002 ==
  BC : BusCreator  Inputs=19
  spec_CnvSet_etaCurr : FromWorkspace  VariableName=testSig_CnvSet_etaCurr  Interpolate=off  OutputAfterFinalValue=Holding final value
  spec_CnvSet_etaCurrNxt : FromWorkspace  VariableName=testSig_CnvSet_etaCurrNxt  Interpolate=off  OutputAfterFinalValue=Holding final value
  spec_CnvSet_etaCurrRmp : FromWorkspace  VariableName=testSig_CnvSet_etaCurrRmp  Interpolate=off  OutputAfterFinalValue=Holding final value
  spec_CnvSet_facRmpVal : FromWorkspace  VariableName=testSig_CnvSet_facRmpVal  Interpolate=off  OutputAfterFinalValue=Holding final value
  spec_CnvSet_qSet : FromWorkspace  VariableName=testSig_CnvSet_qSet  Interpolate=off  OutputAfterFinalValue=Holding final value
  spec_CnvSet_qSetNxt : FromWorkspace  VariableName=testSig_CnvSet_qSetNxt  Interpolate=off  OutputAfterFinalValue=Holding final value
  spec_CnvSet_qSetPrs : FromWorkspace  VariableName=testSig_CnvSet_qSetPrs  Interpolate=off  OutputAfterFinalValue=Holding final value
  spec_CnvSet_qStrt : FromWorkspace  VariableName=testSig_CnvSet_qStrt  Interpolate=off  OutputAfterFinalValue=Holding final value
  spec_CoEOM_facRmpVal : FromWorkspace  VariableName=testSig_CoEOM_facRmpVal  Interpolate=off  OutputAfterFinalValue=Holding final value
  spec_CoEng_stShutOffPath : FromWorkspace  VariableName=testSig_CoEng_stShutOffPath  Interpolate=off  OutputAfterFinalValue=Holding final value
  spec_Epm_nEng : FromWorkspace  VariableName=testSig_Epm_nEng  Interpolate=off  OutputAfterFinalValue=Holding final value
  spec_PhyMod_facEtaCor : FromWorkspace  VariableName=testSig_PhyMod_facEtaCor  Interpolate=off  OutputAfterFinalValue=Holding final value
  spec_PhyMod_facEtaCorNxt : FromWorkspace  VariableName=testSig_PhyMod_facEtaCorNxt  Interpolate=off  OutputAfterFinalValue=Holding final value
  spec_PhyMod_qCor : FromWorkspace  VariableName=testSig_PhyMod_qCor  Interpolate=off  OutputAfterFinalValue=Holding final value
  spec_PhyMod_stNxt : FromWorkspace  VariableName=testSig_PhyMod_stNxt  Interpolate=off  OutputAfterFinalValue=Holding final value
  spec_PhyMod_stPrs : FromWorkspace  VariableName=testSig_PhyMod_stPrs  Interpolate=off  OutputAfterFinalValue=Holding final value
  spec_PthSet_trqInrSet : FromWorkspace  VariableName=testSig_PthSet_trqInrSet  Interpolate=off  OutputAfterFinalValue=Holding final value
  spec_PthSet_trqInrSetAct : FromWorkspace  VariableName=testSig_PthSet_trqInrSetAct  Interpolate=off  OutputAfterFinalValue=Holding final value
  spec_StSys_trqStrt : FromWorkspace  VariableName=testSig_StSys_trqStrt  Interpolate=off  OutputAfterFinalValue=Holding final value
  testSignals : Outport
  wires:
  BC/1 -> testSignals/1
  spec_PthSet_trqInrSet/1 -> BC/1  "testSig_PthSet_trqInrSet"
  spec_StSys_trqStrt/1 -> BC/2  "testSig_StSys_trqStrt"
  spec_Epm_nEng/1 -> BC/3  "testSig_Epm_nEng"
  spec_CoEng_stShutOffPath/1 -> BC/4  "testSig_CoEng_stShutOffPath"
  spec_PhyMod_facEtaCor/1 -> BC/5  "testSig_PhyMod_facEtaCor"
  spec_PhyMod_facEtaCorNxt/1 -> BC/6  "testSig_PhyMod_facEtaCorNxt"
  spec_PhyMod_qCor/1 -> BC/7  "testSig_PhyMod_qCor"
  spec_PhyMod_stPrs/1 -> BC/8  "testSig_PhyMod_stPrs"
  spec_PhyMod_stNxt/1 -> BC/9  "testSig_PhyMod_stNxt"
  spec_CoEOM_facRmpVal/1 -> BC/10  "testSig_CoEOM_facRmpVal"
  spec_CnvSet_qSetPrs/1 -> BC/11  "testSig_CnvSet_qSetPrs"
  spec_CnvSet_etaCurrRmp/1 -> BC/12  "testSig_CnvSet_etaCurrRmp"
  spec_CnvSet_qSet/1 -> BC/13  "testSig_CnvSet_qSet"
  spec_CnvSet_qSetNxt/1 -> BC/14  "testSig_CnvSet_qSetNxt"
  spec_CnvSet_qStrt/1 -> BC/15  "testSig_CnvSet_qStrt"
  spec_CnvSet_facRmpVal/1 -> BC/16  "testSig_CnvSet_facRmpVal"
  spec_CnvSet_etaCurr/1 -> BC/17  "testSig_CnvSet_etaCurr"
  spec_CnvSet_etaCurrNxt/1 -> BC/18  "testSig_CnvSet_etaCurrNxt"
  spec_PthSet_trqInrSetAct/1 -> BC/19  "testSig_PthSet_trqInrSetAct"

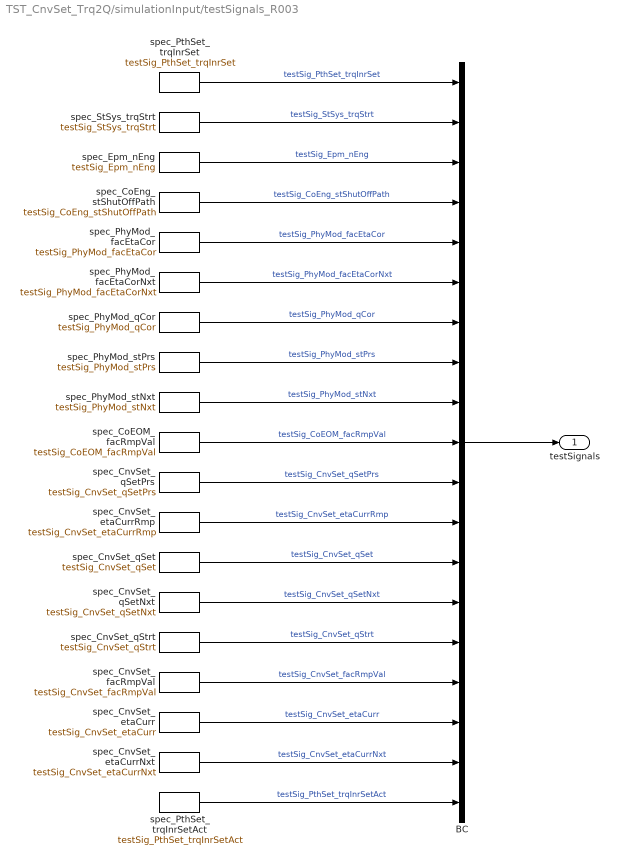
== system TST_CnvSet_Trq2Q/simulationInput/testSignals_R003 ==
  BC : BusCreator  Inputs=19
  spec_CnvSet_etaCurr : FromWorkspace  VariableName=testSig_CnvSet_etaCurr  Interpolate=off  OutputAfterFinalValue=Holding final value
  spec_CnvSet_etaCurrNxt : FromWorkspace  VariableName=testSig_CnvSet_etaCurrNxt  Interpolate=off  OutputAfterFinalValue=Holding final value
  spec_CnvSet_etaCurrRmp : FromWorkspace  VariableName=testSig_CnvSet_etaCurrRmp  Interpolate=off  OutputAfterFinalValue=Holding final value
  spec_CnvSet_facRmpVal : FromWorkspace  VariableName=testSig_CnvSet_facRmpVal  Interpolate=off  OutputAfterFinalValue=Holding final value
  spec_CnvSet_qSet : FromWorkspace  VariableName=testSig_CnvSet_qSet  Interpolate=off  OutputAfterFinalValue=Holding final value
  spec_CnvSet_qSetNxt : FromWorkspace  VariableName=testSig_CnvSet_qSetNxt  Interpolate=off  OutputAfterFinalValue=Holding final value
  spec_CnvSet_qSetPrs : FromWorkspace  VariableName=testSig_CnvSet_qSetPrs  Interpolate=off  OutputAfterFinalValue=Holding final value
  spec_CnvSet_qStrt : FromWorkspace  VariableName=testSig_CnvSet_qStrt  Interpolate=off  OutputAfterFinalValue=Holding final value
  spec_CoEOM_facRmpVal : FromWorkspace  VariableName=testSig_CoEOM_facRmpVal  Interpolate=off  OutputAfterFinalValue=Holding final value
  spec_CoEng_stShutOffPath : FromWorkspace  VariableName=testSig_CoEng_stShutOffPath  Interpolate=off  OutputAfterFinalValue=Holding final value
  spec_Epm_nEng : FromWorkspace  VariableName=testSig_Epm_nEng  Interpolate=off  OutputAfterFinalValue=Holding final value
  spec_PhyMod_facEtaCor : FromWorkspace  VariableName=testSig_PhyMod_facEtaCor  Interpolate=off  OutputAfterFinalValue=Holding final value
  spec_PhyMod_facEtaCorNxt : FromWorkspace  VariableName=testSig_PhyMod_facEtaCorNxt  Interpolate=off  OutputAfterFinalValue=Holding final value
  spec_PhyMod_qCor : FromWorkspace  VariableName=testSig_PhyMod_qCor  Interpolate=off  OutputAfterFinalValue=Holding final value
  spec_PhyMod_stNxt : FromWorkspace  VariableName=testSig_PhyMod_stNxt  Interpolate=off  OutputAfterFinalValue=Holding final value
  spec_PhyMod_stPrs : FromWorkspace  VariableName=testSig_PhyMod_stPrs  Interpolate=off  OutputAfterFinalValue=Holding final value
  spec_PthSet_trqInrSet : FromWorkspace  VariableName=testSig_PthSet_trqInrSet  Interpolate=off  OutputAfterFinalValue=Holding final value
  spec_PthSet_trqInrSetAct : FromWorkspace  VariableName=testSig_PthSet_trqInrSetAct  Interpolate=off  OutputAfterFinalValue=Holding final value
  spec_StSys_trqStrt : FromWorkspace  VariableName=testSig_StSys_trqStrt  Interpolate=off  OutputAfterFinalValue=Holding final value
  testSignals : Outport
  wires:
  BC/1 -> testSignals/1
  spec_PthSet_trqInrSet/1 -> BC/1  "testSig_PthSet_trqInrSet"
  spec_StSys_trqStrt/1 -> BC/2  "testSig_StSys_trqStrt"
  spec_Epm_nEng/1 -> BC/3  "testSig_Epm_nEng"
  spec_CoEng_stShutOffPath/1 -> BC/4  "testSig_CoEng_stShutOffPath"
  spec_PhyMod_facEtaCor/1 -> BC/5  "testSig_PhyMod_facEtaCor"
  spec_PhyMod_facEtaCorNxt/1 -> BC/6  "testSig_PhyMod_facEtaCorNxt"
  spec_PhyMod_qCor/1 -> BC/7  "testSig_PhyMod_qCor"
  spec_PhyMod_stPrs/1 -> BC/8  "testSig_PhyMod_stPrs"
  spec_PhyMod_stNxt/1 -> BC/9  "testSig_PhyMod_stNxt"
  spec_CoEOM_facRmpVal/1 -> BC/10  "testSig_CoEOM_facRmpVal"
  spec_CnvSet_qSetPrs/1 -> BC/11  "testSig_CnvSet_qSetPrs"
  spec_CnvSet_etaCurrRmp/1 -> BC/12  "testSig_CnvSet_etaCurrRmp"
  spec_CnvSet_qSet/1 -> BC/13  "testSig_CnvSet_qSet"
  spec_CnvSet_qSetNxt/1 -> BC/14  "testSig_CnvSet_qSetNxt"
  spec_CnvSet_qStrt/1 -> BC/15  "testSig_CnvSet_qStrt"
  spec_CnvSet_facRmpVal/1 -> BC/16  "testSig_CnvSet_facRmpVal"
  spec_CnvSet_etaCurr/1 -> BC/17  "testSig_CnvSet_etaCurr"
  spec_CnvSet_etaCurrNxt/1 -> BC/18  "testSig_CnvSet_etaCurrNxt"
  spec_PthSet_trqInrSetAct/1 -> BC/19  "testSig_PthSet_trqInrSetAct"

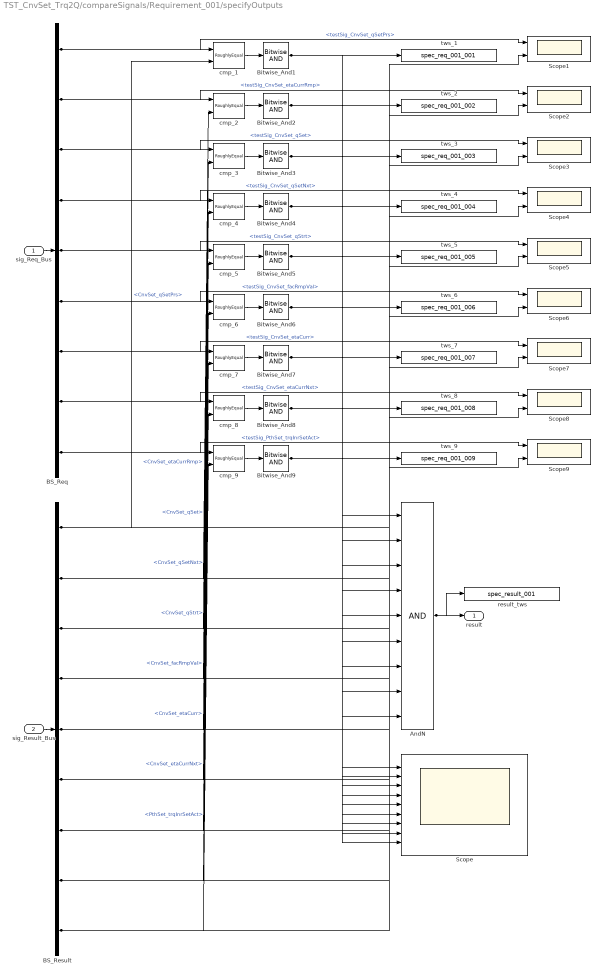
== system TST_CnvSet_Trq2Q/compareSignals/Requirement_001/specifyOutputs ==
  sig_Req_Bus : Inport
  sig_Result_Bus : Inport  Port=2
  AndN : Logic  Inputs=9
  BS_Req : BusSelector  OutputSignals=testSig_CnvSet_qSetPrs,testSig_CnvSet_etaCurrRmp,testSig_CnvSet_qSet,testSig_CnvSet_qSetNxt,testSig_CnvSet_qStrt,testSig_CnvSet_facRmpVal,testSig_CnvSet_etaCurr,testSig_CnvSet_etaCurrNxt,testSig_PthSet_trqInrSetAct
  BS_Result : BusSelector  OutputSignals=CnvSet_qSetPrs,CnvSet_etaCurrRmp,CnvSet_qSet,CnvSet_qSetNxt,CnvSet_qStrt,CnvSet_facRmpVal,CnvSet_etaCurr,CnvSet_etaCurrNxt,PthSet_trqInrSetAct
  Bitwise_And{1..9} (9 alike) : simulink/Logic and Bit Operations/Bitwise Operator  logicop=AND  UseBitMask=off  BitMask=bin2dec('11011001')  BitMaskRealWorld=Stored Integer
  Scope : Scope  NumInputPorts=9
  Scope{1..9} (9 alike) : Scope  NumInputPorts=2
  cmp_{1..9} (9 alike) : UnitTest_Lib/RoughlyEqual  slope=0.1
  result_tws : ToWorkspace  VariableName=spec_result_001
  tws_1 : ToWorkspace  VariableName=spec_req_001_001
  tws_2 : ToWorkspace  VariableName=spec_req_001_002
  tws_3 : ToWorkspace  VariableName=spec_req_001_003
  tws_4 : ToWorkspace  VariableName=spec_req_001_004
  tws_5 : ToWorkspace  VariableName=spec_req_001_005
  tws_6 : ToWorkspace  VariableName=spec_req_001_006
  tws_7 : ToWorkspace  VariableName=spec_req_001_007
  tws_8 : ToWorkspace  VariableName=spec_req_001_008
  tws_9 : ToWorkspace  VariableName=spec_req_001_009
  result : Outport
  wires:
  sig_Req_Bus/1 -> BS_Req/1
  sig_Result_Bus/1 -> BS_Result/1
  AndN/1 -> result/1, result_tws/1
  BS_Req/1 -> cmp_1/1, Scope1/1  "<testSig_CnvSet_qSetPrs>"
  BS_Result/1 -> cmp_1/2, Scope1/2  "<CnvSet_qSetPrs>"
  cmp_1/1 -> Bitwise_And1/1
  Bitwise_And1/1 -> tws_1/1, AndN/1, Scope/1
  BS_Req/2 -> cmp_2/1, Scope2/1  "<testSig_CnvSet_etaCurrRmp>"
  BS_Result/2 -> cmp_2/2, Scope2/2  "<CnvSet_etaCurrRmp>"
  cmp_2/1 -> Bitwise_And2/1
  Bitwise_And2/1 -> tws_2/1, AndN/2, Scope/2
  BS_Req/3 -> cmp_3/1, Scope3/1  "<testSig_CnvSet_qSet>"
  BS_Result/3 -> cmp_3/2, Scope3/2  "<CnvSet_qSet>"
  cmp_3/1 -> Bitwise_And3/1
  Bitwise_And3/1 -> tws_3/1, AndN/3, Scope/3
  BS_Req/4 -> cmp_4/1, Scope4/1  "<testSig_CnvSet_qSetNxt>"
  BS_Result/4 -> cmp_4/2, Scope4/2  "<CnvSet_qSetNxt>"
  cmp_4/1 -> Bitwise_And4/1
  Bitwise_And4/1 -> tws_4/1, AndN/4, Scope/4
  BS_Req/5 -> cmp_5/1, Scope5/1  "<testSig_CnvSet_qStrt>"
  BS_Result/5 -> cmp_5/2, Scope5/2  "<CnvSet_qStrt>"
  cmp_5/1 -> Bitwise_And5/1
  Bitwise_And5/1 -> tws_5/1, AndN/5, Scope/5
  BS_Req/6 -> cmp_6/1, Scope6/1  "<testSig_CnvSet_facRmpVal>"
  BS_Result/6 -> cmp_6/2, Scope6/2  "<CnvSet_facRmpVal>"
  cmp_6/1 -> Bitwise_And6/1
  Bitwise_And6/1 -> tws_6/1, AndN/6, Scope/6
  BS_Req/7 -> cmp_7/1, Scope7/1  "<testSig_CnvSet_etaCurr>"
  BS_Result/7 -> cmp_7/2, Scope7/2  "<CnvSet_etaCurr>"
  cmp_7/1 -> Bitwise_And7/1
  Bitwise_And7/1 -> tws_7/1, AndN/7, Scope/7
  BS_Req/8 -> cmp_8/1, Scope8/1  "<testSig_CnvSet_etaCurrNxt>"
  BS_Result/8 -> cmp_8/2, Scope8/2  "<CnvSet_etaCurrNxt>"
  cmp_8/1 -> Bitwise_And8/1
  Bitwise_And8/1 -> tws_8/1, AndN/8, Scope/8
  BS_Req/9 -> cmp_9/1, Scope9/1  "<testSig_PthSet_trqInrSetAct>"
  BS_Result/9 -> cmp_9/2, Scope9/2  "<PthSet_trqInrSetAct>"
  cmp_9/1 -> Bitwise_And9/1
  Bitwise_And9/1 -> tws_9/1, AndN/9, Scope/9

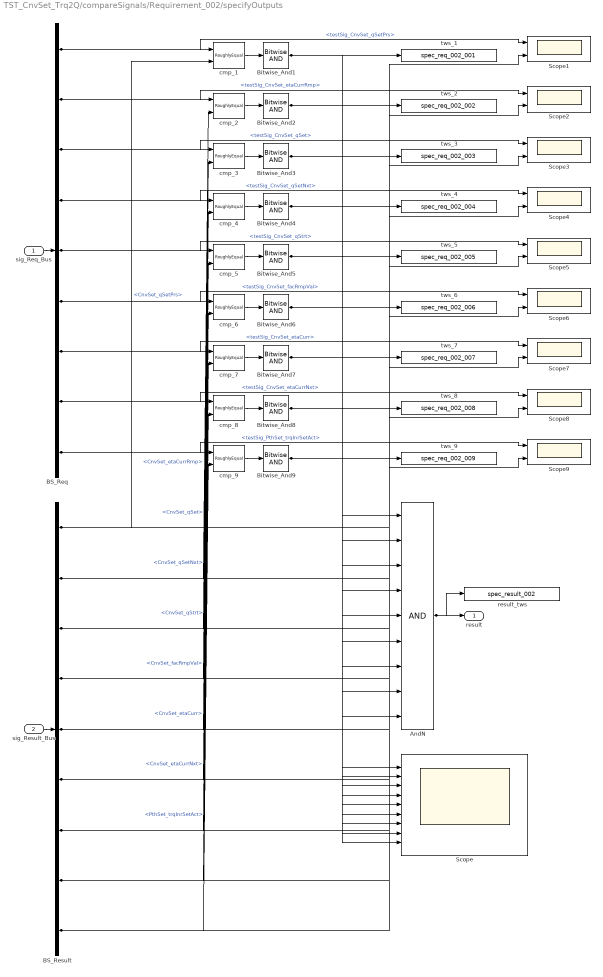
== system TST_CnvSet_Trq2Q/compareSignals/Requirement_002/specifyOutputs ==
  sig_Req_Bus : Inport
  sig_Result_Bus : Inport  Port=2
  AndN : Logic  Inputs=9
  BS_Req : BusSelector  OutputSignals=testSig_CnvSet_qSetPrs,testSig_CnvSet_etaCurrRmp,testSig_CnvSet_qSet,testSig_CnvSet_qSetNxt,testSig_CnvSet_qStrt,testSig_CnvSet_facRmpVal,testSig_CnvSet_etaCurr,testSig_CnvSet_etaCurrNxt,testSig_PthSet_trqInrSetAct
  BS_Result : BusSelector  OutputSignals=CnvSet_qSetPrs,CnvSet_etaCurrRmp,CnvSet_qSet,CnvSet_qSetNxt,CnvSet_qStrt,CnvSet_facRmpVal,CnvSet_etaCurr,CnvSet_etaCurrNxt,PthSet_trqInrSetAct
  Bitwise_And{1..9} (9 alike) : simulink/Logic and Bit Operations/Bitwise Operator  logicop=AND  UseBitMask=off  BitMask=bin2dec('11011001')  BitMaskRealWorld=Stored Integer
  Scope : Scope  NumInputPorts=9
  Scope{1..9} (9 alike) : Scope  NumInputPorts=2
  cmp_{1..9} (9 alike) : UnitTest_Lib/RoughlyEqual  slope=0.1
  result_tws : ToWorkspace  VariableName=spec_result_002
  tws_1 : ToWorkspace  VariableName=spec_req_002_001
  tws_2 : ToWorkspace  VariableName=spec_req_002_002
  tws_3 : ToWorkspace  VariableName=spec_req_002_003
  tws_4 : ToWorkspace  VariableName=spec_req_002_004
  tws_5 : ToWorkspace  VariableName=spec_req_002_005
  tws_6 : ToWorkspace  VariableName=spec_req_002_006
  tws_7 : ToWorkspace  VariableName=spec_req_002_007
  tws_8 : ToWorkspace  VariableName=spec_req_002_008
  tws_9 : ToWorkspace  VariableName=spec_req_002_009
  result : Outport
  wires:
  sig_Req_Bus/1 -> BS_Req/1
  sig_Result_Bus/1 -> BS_Result/1
  AndN/1 -> result/1, result_tws/1
  BS_Req/1 -> cmp_1/1, Scope1/1  "<testSig_CnvSet_qSetPrs>"
  BS_Result/1 -> cmp_1/2, Scope1/2  "<CnvSet_qSetPrs>"
  cmp_1/1 -> Bitwise_And1/1
  Bitwise_And1/1 -> tws_1/1, AndN/1, Scope/1
  BS_Req/2 -> cmp_2/1, Scope2/1  "<testSig_CnvSet_etaCurrRmp>"
  BS_Result/2 -> cmp_2/2, Scope2/2  "<CnvSet_etaCurrRmp>"
  cmp_2/1 -> Bitwise_And2/1
  Bitwise_And2/1 -> tws_2/1, AndN/2, Scope/2
  BS_Req/3 -> cmp_3/1, Scope3/1  "<testSig_CnvSet_qSet>"
  BS_Result/3 -> cmp_3/2, Scope3/2  "<CnvSet_qSet>"
  cmp_3/1 -> Bitwise_And3/1
  Bitwise_And3/1 -> tws_3/1, AndN/3, Scope/3
  BS_Req/4 -> cmp_4/1, Scope4/1  "<testSig_CnvSet_qSetNxt>"
  BS_Result/4 -> cmp_4/2, Scope4/2  "<CnvSet_qSetNxt>"
  cmp_4/1 -> Bitwise_And4/1
  Bitwise_And4/1 -> tws_4/1, AndN/4, Scope/4
  BS_Req/5 -> cmp_5/1, Scope5/1  "<testSig_CnvSet_qStrt>"
  BS_Result/5 -> cmp_5/2, Scope5/2  "<CnvSet_qStrt>"
  cmp_5/1 -> Bitwise_And5/1
  Bitwise_And5/1 -> tws_5/1, AndN/5, Scope/5
  BS_Req/6 -> cmp_6/1, Scope6/1  "<testSig_CnvSet_facRmpVal>"
  BS_Result/6 -> cmp_6/2, Scope6/2  "<CnvSet_facRmpVal>"
  cmp_6/1 -> Bitwise_And6/1
  Bitwise_And6/1 -> tws_6/1, AndN/6, Scope/6
  BS_Req/7 -> cmp_7/1, Scope7/1  "<testSig_CnvSet_etaCurr>"
  BS_Result/7 -> cmp_7/2, Scope7/2  "<CnvSet_etaCurr>"
  cmp_7/1 -> Bitwise_And7/1
  Bitwise_And7/1 -> tws_7/1, AndN/7, Scope/7
  BS_Req/8 -> cmp_8/1, Scope8/1  "<testSig_CnvSet_etaCurrNxt>"
  BS_Result/8 -> cmp_8/2, Scope8/2  "<CnvSet_etaCurrNxt>"
  cmp_8/1 -> Bitwise_And8/1
  Bitwise_And8/1 -> tws_8/1, AndN/8, Scope/8
  BS_Req/9 -> cmp_9/1, Scope9/1  "<testSig_PthSet_trqInrSetAct>"
  BS_Result/9 -> cmp_9/2, Scope9/2  "<PthSet_trqInrSetAct>"
  cmp_9/1 -> Bitwise_And9/1
  Bitwise_And9/1 -> tws_9/1, AndN/9, Scope/9

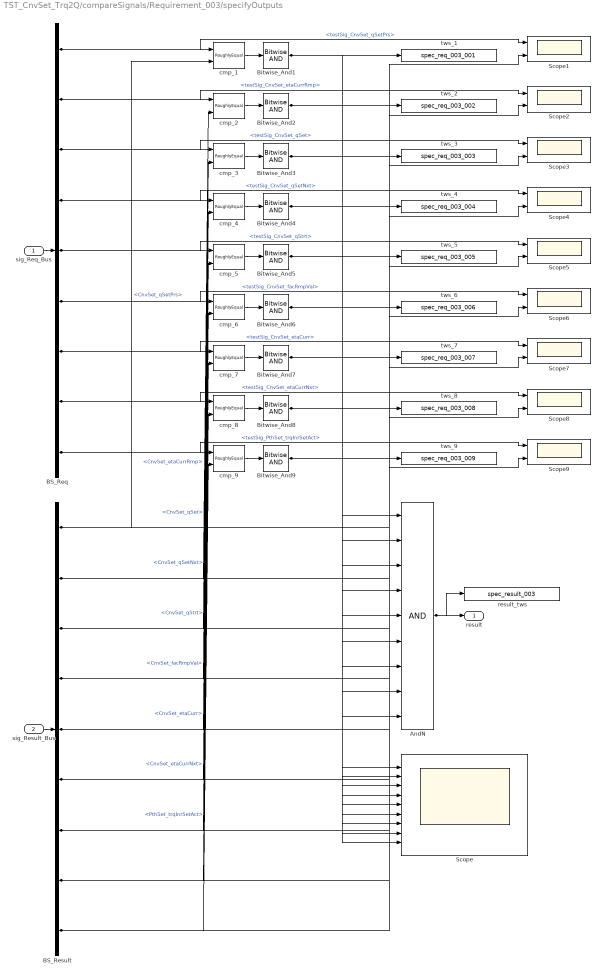
== system TST_CnvSet_Trq2Q/compareSignals/Requirement_003/specifyOutputs ==
  sig_Req_Bus : Inport
  sig_Result_Bus : Inport  Port=2
  AndN : Logic  Inputs=9
  BS_Req : BusSelector  OutputSignals=testSig_CnvSet_qSetPrs,testSig_CnvSet_etaCurrRmp,testSig_CnvSet_qSet,testSig_CnvSet_qSetNxt,testSig_CnvSet_qStrt,testSig_CnvSet_facRmpVal,testSig_CnvSet_etaCurr,testSig_CnvSet_etaCurrNxt,testSig_PthSet_trqInrSetAct
  BS_Result : BusSelector  OutputSignals=CnvSet_qSetPrs,CnvSet_etaCurrRmp,CnvSet_qSet,CnvSet_qSetNxt,CnvSet_qStrt,CnvSet_facRmpVal,CnvSet_etaCurr,CnvSet_etaCurrNxt,PthSet_trqInrSetAct
  Bitwise_And{1..9} (9 alike) : simulink/Logic and Bit Operations/Bitwise Operator  logicop=AND  UseBitMask=off  BitMask=bin2dec('11011001')  BitMaskRealWorld=Stored Integer
  Scope : Scope  NumInputPorts=9
  Scope{1..9} (9 alike) : Scope  NumInputPorts=2
  cmp_{1..9} (9 alike) : UnitTest_Lib/RoughlyEqual  slope=0.1
  result_tws : ToWorkspace  VariableName=spec_result_003
  tws_1 : ToWorkspace  VariableName=spec_req_003_001
  tws_2 : ToWorkspace  VariableName=spec_req_003_002
  tws_3 : ToWorkspace  VariableName=spec_req_003_003
  tws_4 : ToWorkspace  VariableName=spec_req_003_004
  tws_5 : ToWorkspace  VariableName=spec_req_003_005
  tws_6 : ToWorkspace  VariableName=spec_req_003_006
  tws_7 : ToWorkspace  VariableName=spec_req_003_007
  tws_8 : ToWorkspace  VariableName=spec_req_003_008
  tws_9 : ToWorkspace  VariableName=spec_req_003_009
  result : Outport
  wires:
  sig_Req_Bus/1 -> BS_Req/1
  sig_Result_Bus/1 -> BS_Result/1
  AndN/1 -> result/1, result_tws/1
  BS_Req/1 -> cmp_1/1, Scope1/1  "<testSig_CnvSet_qSetPrs>"
  BS_Result/1 -> cmp_1/2, Scope1/2  "<CnvSet_qSetPrs>"
  cmp_1/1 -> Bitwise_And1/1
  Bitwise_And1/1 -> tws_1/1, AndN/1, Scope/1
  BS_Req/2 -> cmp_2/1, Scope2/1  "<testSig_CnvSet_etaCurrRmp>"
  BS_Result/2 -> cmp_2/2, Scope2/2  "<CnvSet_etaCurrRmp>"
  cmp_2/1 -> Bitwise_And2/1
  Bitwise_And2/1 -> tws_2/1, AndN/2, Scope/2
  BS_Req/3 -> cmp_3/1, Scope3/1  "<testSig_CnvSet_qSet>"
  BS_Result/3 -> cmp_3/2, Scope3/2  "<CnvSet_qSet>"
  cmp_3/1 -> Bitwise_And3/1
  Bitwise_And3/1 -> tws_3/1, AndN/3, Scope/3
  BS_Req/4 -> cmp_4/1, Scope4/1  "<testSig_CnvSet_qSetNxt>"
  BS_Result/4 -> cmp_4/2, Scope4/2  "<CnvSet_qSetNxt>"
  cmp_4/1 -> Bitwise_And4/1
  Bitwise_And4/1 -> tws_4/1, AndN/4, Scope/4
  BS_Req/5 -> cmp_5/1, Scope5/1  "<testSig_CnvSet_qStrt>"
  BS_Result/5 -> cmp_5/2, Scope5/2  "<CnvSet_qStrt>"
  cmp_5/1 -> Bitwise_And5/1
  Bitwise_And5/1 -> tws_5/1, AndN/5, Scope/5
  BS_Req/6 -> cmp_6/1, Scope6/1  "<testSig_CnvSet_facRmpVal>"
  BS_Result/6 -> cmp_6/2, Scope6/2  "<CnvSet_facRmpVal>"
  cmp_6/1 -> Bitwise_And6/1
  Bitwise_And6/1 -> tws_6/1, AndN/6, Scope/6
  BS_Req/7 -> cmp_7/1, Scope7/1  "<testSig_CnvSet_etaCurr>"
  BS_Result/7 -> cmp_7/2, Scope7/2  "<CnvSet_etaCurr>"
  cmp_7/1 -> Bitwise_And7/1
  Bitwise_And7/1 -> tws_7/1, AndN/7, Scope/7
  BS_Req/8 -> cmp_8/1, Scope8/1  "<testSig_CnvSet_etaCurrNxt>"
  BS_Result/8 -> cmp_8/2, Scope8/2  "<CnvSet_etaCurrNxt>"
  cmp_8/1 -> Bitwise_And8/1
  Bitwise_And8/1 -> tws_8/1, AndN/8, Scope/8
  BS_Req/9 -> cmp_9/1, Scope9/1  "<testSig_PthSet_trqInrSetAct>"
  BS_Result/9 -> cmp_9/2, Scope9/2  "<PthSet_trqInrSetAct>"
  cmp_9/1 -> Bitwise_And9/1
  Bitwise_And9/1 -> tws_9/1, AndN/9, Scope/9
